simulink model "HCU_V2_Simulink"  (R2025b)
settings: Solver=FixedStepDiscrete  StartTime=0.0  StopTime=10.0  FixedStep=0.01  RelTol=1e-3
libraries: simulink x30, hdlsllib x9, etargetslib x7
(part 2 of 2)

== stateflow chart HCU_V2_Simulink/Logic/Safety_Supervisor ==
  state VALIDATING_FAULT_FROM_STANDBY
  state HV_OFF
    entry:
    AIR_Enable = false;
    Pre_Charge_Enable = false;
    Inverter_Enable = false;
    State_Enum = 1;
    Fault_Cause = 0;
    Fault_Code = 0;
  state PRE_CHARGE
    entry:
    Pre_Charge_Enable = true;
    State_Enum = 3;
  state RELAY_SWAP
    entry:
    Pre_Charge_Enable = true;
    AIR_Enable = true;
    State_Enum = 4;
  state DRIVE
    entry:
    AIR_Enable = true;
    Pre_Charge_Enable = false;
    Inverter_Enable = true;
    State_Enum = 5;
  state STANDBY
    entry:
    State_Enum = 2;
  state VALIDATING_ERROR_STATE1
  state VALIDATING_ERROR_STATE
  state VALIDATING_ERROR_STATE3
  state VALIDATING_ERROR_STATE2
  state VALIDATING_ERROR_STATE4
  state Error_State
    entry:
    Fault_Code = Fault_Cause;
    AIR_Enable = false;
    Pre_Charge_Enable = false;
    Inverter_Enable = false;
    State_Enum = 6;
  state VALIDATING_APPS_IMPLAUSIBILITY
  DRIVE -> HV_OFF [order 3] : [~SDC_Monitor]
  RELAY_SWAP -> HV_OFF [order 3] : [~SDC_Monitor]
  PRE_CHARGE -> HV_OFF [order 4] : [~SDC_Monitor]
  STANDBY -> VALIDATING_FAULT_FROM_STANDBY [order 2] : [APPS_Implausibility]
  VALIDATING_FAULT_FROM_STANDBY -> HV_OFF [order 1] : after(0.1,sec)
  VALIDATING_FAULT_FROM_STANDBY -> STANDBY [order 2] : [~APPS_Implausibility]
  PRE_CHARGE -> RELAY_SWAP [order 1] : [Bus_Voltage_FL > (0.9 * Voltage) && Bus_Voltage_FR > (0.9 * Voltage)]
  RELAY_SWAP -> DRIVE [order 1] : after(100, msec)
  STANDBY -> PRE_CHARGE [order 1] : [Brake_Pressure > 10 && Start_Button && Synced]
  HV_OFF -> STANDBY [order 1] : [~BMS_Fault]
  VALIDATING_ERROR_STATE3 -> STANDBY [order 1] : [~BMS_Fault]
  VALIDATING_ERROR_STATE -> PRE_CHARGE [order 2] : [~BMS_Fault]
  (default) -> HV_OFF
  STANDBY -> HV_OFF [order 4] : [~SDC_Monitor]
  STANDBY -> VALIDATING_ERROR_STATE3 [order 3] : [BMS_Fault]{Fault_Cause = 20;}
  PRE_CHARGE -> Error_State [order 2] : after(3,sec){Fault_Cause = 40;}
  PRE_CHARGE -> VALIDATING_ERROR_STATE [order 3] : [BMS_Fault]{Fault_Cause = 20;}
  VALIDATING_ERROR_STATE1 -> RELAY_SWAP [order 2] : [~BMS_Fault]
  RELAY_SWAP -> VALIDATING_ERROR_STATE1 [order 2] : [BMS_Fault]{Fault_Cause = 20;}
  VALIDATING_APPS_IMPLAUSIBILITY -> DRIVE [order 1] : [~APPS_Implausibility]
  DRIVE -> VALIDATING_APPS_IMPLAUSIBILITY [order 2] : [APPS_Implausibility]
  DRIVE -> VALIDATING_ERROR_STATE2 [order 1] : [BMS_Fault]{Fault_Cause = 20;}
  VALIDATING_ERROR_STATE2 -> DRIVE [order 1] : [~BMS_Fault]
  Error_State -> HV_OFF : [ resetReq && ~BMS_Fault ] { Fault_Code = 0; Fault_Cause = 0; }
  VALIDATING_APPS_IMPLAUSIBILITY -> HV_OFF [order 2] : after(100,msec)
  HV_OFF -> VALIDATING_ERROR_STATE4 [order 2] : [BMS_Fault]{Fault_Cause = 20;}
  VALIDATING_ERROR_STATE4 -> HV_OFF [order 1] : [~BMS_Fault]
  VALIDATING_ERROR_STATE1 -> Error_State [order 1] : after(100,msec)
  VALIDATING_ERROR_STATE -> Error_State [order 1] : after(100,msec)
  VALIDATING_ERROR_STATE3 -> Error_State [order 2] : after(100,msec)
  VALIDATING_ERROR_STATE2 -> Error_State [order 2] : after(100,msec)
  VALIDATING_ERROR_STATE4 -> Error_State [order 2] : after(100,msec)
  data: Voltage input single size=1; APPS_Implausibility input; BMS_Fault input; Synced input boolean; Brake_Pressure input; Start_Button input; AIR_Enable output boolean; Inverter_Enable output boolean; Pre_Charge_Enable output; Bus_Voltage_FL input; Bus_Voltage_FR input; SDC_Monitor input; State_Enum output uint8; Fault_Code output uint8; Fault_Cause local uint8; resetReq input

== matlab function HCU_V2_Simulink/Encoder_Velocity_Decode/MATLAB Function ==
  data: CAN_Data input; Vel_Estimate output
function Vel_Estimate = decode_vel(CAN_Data)
    d = uint8(CAN_Data(:));    % 8x1 uint8, orientation-proof
    % bytes 4-7, little-endian: byte4 = LSB ... byte7 = MSB (bytes 0-3 ignored)
    v = bitor(bitor(           uint32(d(5)),      bitshift(uint32(d(6)),  8)), ...
              bitor(bitshift(uint32(d(7)), 16),   bitshift(uint32(d(8)), 24)));
    Vel_Estimate = typecast(v, 'single');   % scalar uint32 -> scalar single (1x1), turns/s
end

== matlab function HCU_V2_Simulink/Encoder_Velocity_Decode/MATLAB Function1 ==
  data: CAN_Data input; Vel_Estimate output
function Vel_Estimate = decode_vel(CAN_Data)
    d = uint8(CAN_Data(:));    % 8x1 uint8, orientation-proof
    % bytes 4-7, little-endian: byte4 = LSB ... byte7 = MSB (bytes 0-3 ignored)
    v = bitor(bitor(           uint32(d(5)),      bitshift(uint32(d(6)),  8)), ...
              bitor(bitshift(uint32(d(7)), 16),   bitshift(uint32(d(8)), 24)));
    Vel_Estimate = typecast(v, 'single');   % scalar uint32 -> scalar single (1x1), turns/s
end

== matlab function HCU_V2_Simulink/Logic/Torque_Power_Limiter ==
  data: tauL_req input; tauL_cmd output; tauR_req input; velL input; velR input; velL_age input; velR_age input; dcl input; acl input; vpack input; bms_age input; drive_eff input; regen_eff input; bms_margin input; motor_torque_max input; tauR_cmd output; s output; p_demand output; p_budget output; motor_regen_max input; regen_cutoff_speed input
function [tauL_cmd, tauR_cmd, s, p_demand, p_budget] = bms_power_limit( ...
        tauL_req, tauR_req, ...                 % SIGNED net torque [Nm] per wheel (drive +, regen -),
        ...                                     %   from YOUR decision blocks (APPS/brake/lookups/TV)
        velL, velR, ...                         % motor speeds [turns/s], unpacked to single
        velL_age, velR_age, ...                 % ms since last seen, uint32
        dcl, acl, vpack, bms_age, ...           % DCL [A], ACL [A], pack V [V], BMS frame age [ms]
        drive_eff, regen_eff, bms_margin, ...   % efficiencies + safety margin
        motor_torque_max, motor_regen_max, ...  % per-wheel caps [Nm], both >=0 magnitudes
        regen_cutoff_speed)                     % low-speed regen taper [turns/s]
%#codegen
% PURE LIMITER. Takes a SIGNED net torque request per wheel and makes it safe.
% NO torque decision here - APPS curves, brake->regen, lookup tables and torque
% vectoring all live UPSTREAM in visible blocks and arrive baked into tau*_req
% (drive = +, regen = -). This block only: caps to motor limits, tapers regen at
% low speed, and scales BOTH wheels by ONE factor s so total pack power stays
% within DCL (discharge) / ACL (charge). Direction multiply + CAN packing stay
% OUTSIDE (unchanged). See memory: bms-torque-limit-strategy.

    % ---- safety constants (deliberately NOT tunable) ----
    MAX_AGE_MS = uint32(150);         % CAN freshness window; older => fault
    EPS_W      = single(1.0);         % floor on |power|, guards the divide
    EPS_DEN    = single(1.0e-3);      % floor on efficiency / cutoff divides
    TWO_PI     = single(6.2831853);   % turns/s -> rad/s. If vel ALREADY rad/s, set 1.0

    % speed MAGNITUDE in rad/s -> mounting sign never matters in the power calc
    wL = TWO_PI * single(abs(velL));
    wR = TWO_PI * single(abs(velR));

    % ---- low-speed taper: fade ONLY the regen (negative) part as |vel| -> 0, so
    % the motor never reverse-drives a stopped car (torque is a HOLDING torque
    % even as power->0). Drive torque is left untouched.
    cutoff = max(single(regen_cutoff_speed), EPS_DEN);
    gL = min(single(1.0), single(abs(velL)) / cutoff);
    gR = min(single(1.0), single(abs(velR)) / cutoff);
    tauL_t = single(tauL_req);
    tauR_t = single(tauR_req);
    if tauL_t < single(0.0)
        tauL_t = tauL_t * gL;
    end
    if tauR_t < single(0.0)
        tauR_t = tauR_t * gR;
    end

    % ---- per-wheel cap [-motor_regen_max, +motor_torque_max] (also stall guard) -
    tauL1 = min(max(tauL_t, -single(motor_regen_max)), single(motor_torque_max));
    tauR1 = min(max(tauR_t, -single(motor_regen_max)), single(motor_torque_max));

    % ---- SIGNED pack power demand [W]: >0 draws from pack, <0 charges it -------
    p_demand = tauL1 * wL + tauR1 * wR;

    % ---- pick the binding budget by power direction (efficiency asymmetry) -----
    % dcl<=0 / acl<=0 / vpack<=0 make p_budget<=0 => s clamps to 0 automatically,
    % so an invalid limit disables only the side that is actually using it.
    if p_demand >= single(0.0)
        % discharge: mech out = eff * elec drawn  => budget *= eff
        p_budget = single(drive_eff) * single(bms_margin) * single(dcl) * single(vpack);
        s = p_budget / max(p_demand, EPS_W);
    else
        % charge:  elec in = eff * mech absorbed  => budget /= eff  (regen_eff ~0.95)
        p_budget = single(bms_margin) * single(acl) * single(vpack) / max(single(regen_eff), EPS_DEN);
        s = p_budget / max(-p_demand, EPS_W);
    end
    s = min(single(1.0), max(single(0.0), s));

    % ---- validity gate (BRAKE freshness is handled UPSTREAM in the decision
    % block - a stale brake => 0 regen there; this gate cuts BOTH on bad BMS/vel) -
    ok = (bms_age  < MAX_AGE_MS) && ...
         (velL_age < MAX_AGE_MS) && ...
         (velR_age < MAX_AGE_MS) && ...
         (vpack > single(0.0));
    if ~ok
        s = single(0.0);
    end

    % ---- limited torque (vehicle frame; Direction multiply + packing outside) --
    tauL_cmd = s * tauL1;
    tauR_cmd = s * tauR1;
end
